simulink model "doc_rscoding"  (R2014a)
settings: Solver=ode45  StartTime=0.0  StopTime=500  RelTol=1e-3
undefined symbols (not defined in the file or in its folder): rsgenpoly
libraries: commblkcod2 x2, simulink x1, commrandsrc2 x1
settings Model: Creator=The MathWorks Inc.
settings DataIOCC: SignalLoggingSaveFormat=ModelDataLogs  SignalLoggingName=logsOut
settings OptimizationCC: BlockReduction=off  BooleanDataType=off  ExpressionDepthLimit=2147483647
settings DebuggingCC: SaveWithParameterizedLinksMsg=none  UnderspecifiedInitializationDetection=Classic  SolverPrmCheckMsg=none  MultiTaskDSMMsg=warning  MultiTaskCondExecSysMsg=none  FcnCallInpInsideContextMsg=UseLocalSettings  StateNameClashWarn=warning  StrictBusMsg=None
settings HardwareCC: ProdHWDeviceType=Specified
settings RTWCC: IncludeERTFirstTime=on
settings CodeAppCC: MangleLength=5
settings GRTTargetCC: TargetFcnLib=iso_c_tmw.mat  CombineOutputUpdateFcns=off  GRTInterface=on

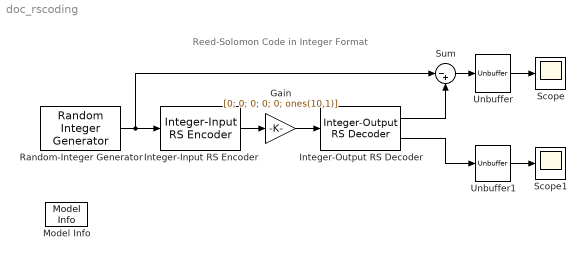
== system doc_rscoding ==
  note: Reed-Solomon Code in Integer Format
  Gain : Gain  Gain=[0; 0; 0; 0; 0; ones(10,1)]  SaturateOnIntegerOverflow=on  OutDataTypeStr=Inherit: Same as input  ParamDataTypeStr=Inherit: Same as input
  Integer-Input RS Encoder : commblkcod2/Integer-Input RS Encoder  n=15  k=5  specPrimPoly=off  prPoly=[1 0 1 1]  specGenPoly=off  genPoly=rsgenpoly(7,3)  specPuncture=off  punctVec=[ones(2,1); zeros(2,1)]
  Integer-Output RS Decoder : commblkcod2/Integer-Output RS Decoder  n=15  k=5  specPrimPoly=off  prPoly=[1 0 1 1]  specGenPoly=off  genPoly=rsgenpoly(7,3)  specPuncture=off  punctVec=[ones(2,1); zeros(2,1)]  specErasurePort=off  showNumErr=on
  Model Info : simulink/Model-Wide Utilities/Model Info  InitialBlockCM=None  BlockCM=none  Frame=on  DisplayStringWithTags=Info  HorizontalTextAlignment=Center  LeftAlignmentValue=0.5  SourceBlockDiagram=doc_rscoding  TagMaxNumber=20
  Random-Integer Generator : commrandsrc2/Random Integer Generator  mul=15  seed=68521  Ts=1  frameBased=on  sampPerFrame=5  orient=off  outDataType=double
  Scope : Scope
  Scope1 : Scope
      settings: YMin=0  YMax=6
  Sum : Sum  Inputs=|-+  SaturateOnIntegerOverflow=on  InputSameDT=on  OutDataTypeStr=Inherit: Same as first input
  Unbuffer : Unbuffer  SampleBasedProcessing=Same as frame based
  Unbuffer1 : Unbuffer  SampleBasedProcessing=Same as frame based
  wires:
  Sum/1 -> Unbuffer/1
  Integer-Input RS Encoder/1 -> Gain/1
  Gain/1 -> Integer-Output RS Decoder/1
  Integer-Output RS Decoder/1 -> Sum/2
  Random-Integer Generator/1 -> Integer-Input RS Encoder/1, Sum/1
  Integer-Output RS Decoder/2 -> Unbuffer1/1
  Unbuffer/1 -> Scope/1
  Unbuffer1/1 -> Scope1/1
